simulink model "sampleModel1599_1"  (R2023a)
settings: Solver=VariableStepAuto  StartTime=0.0  StopTime=10.0  RelTol=1e-3
libraries: hdlsllib x2, simulink x2
settings Model: Creator=user1  LastModifiedBy=user1

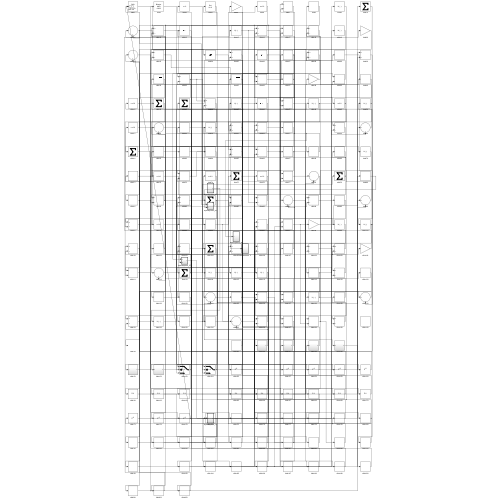
[thumbnail: Simulink's stored preview of the top-level diagram]
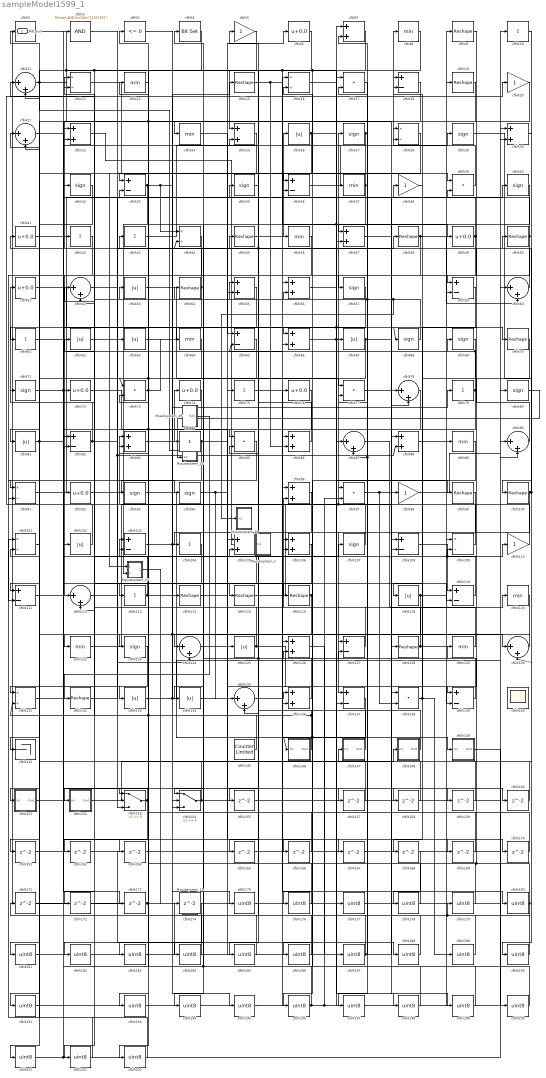
== system sampleModel1599_1 ==
  Mysubsystem_11 : Subsystem  TreatAsAtomicUnit=on  RTWFcnName=Mysubsystem_11
      settings: RTWFcnNameOpts=User specified  RTWFileNameOpts=Use function name
  Mysubsystem_2 : Subsystem  TreatAsAtomicUnit=on  RTWFcnName=Mysubsystem_2
      settings: RTWFcnNameOpts=User specified  RTWFileNameOpts=Use function name
  Mysubsystem_20 : Subsystem  TreatAsAtomicUnit=on  RTWFcnName=Mysubsystem_20
      settings: RTWFcnNameOpts=User specified  RTWFileNameOpts=Use function name
  Mysubsystem_27 : Subsystem  TreatAsAtomicUnit=on  RTWFcnName=Mysubsystem_27
      settings: RTWFcnNameOpts=User specified  RTWFileNameOpts=Use function name
  Mysubsystem_48 : Subsystem  TreatAsAtomicUnit=on  RTWFcnName=Mysubsystem_48
      settings: RTWFcnNameOpts=User specified  RTWFileNameOpts=Use function name
  Mysubsystem_49 : Subsystem  TreatAsAtomicUnit=on  RTWFcnName=Mysubsystem_49
      settings: RTWFcnNameOpts=User specified  RTWFileNameOpts=Use function name
  cfblk1 : ArithShift  BitShiftNumber=8
  cfblk{10,42..43,61,75,79,84,104,113} (9 alike) : Sum  Inputs=+  OutDataTypeStr=uint8
  cfblk{9,15,19,45,48,50,54,70,99..100,114..116,128,132} (15 alike) : Reshape
  cfblk{12,16,28,44,91,101,109,131} (8 alike) : Product  Inputs=*/  OutDataTypeStr=uint8  RndMeth=Zero  SaturateOnIntegerOverflow=on
  cfblk{26,53,62..63,67,81,102,118,125,133..134} (11 alike) : Abs  OutDataTypeStr=uint8  SaturateOnIntegerOverflow=off
  cfblk{18,33,36,59,65,82,103,108,111,119,127,137,139} (13 alike) : Sum  Inputs=+-  OutDataTypeStr=uint8
  cfblk{7,22,25,30,47,55..56,66,83,86,88,96,105..106,126,136} (16 alike) : Sum  OutDataTypeStr=uint8
  cfblk{27,29,32,35,40,57,68..69,71,80,93..94,107,123} (14 alike) : Signum
  cfblk{11,21,52,60,78,87,90,112,124,130,135} (11 alike) : Sum  Inputs=|++  OutDataTypeStr=uint8
  cfblk{5,20,38,98,110} (5 alike) : Gain  OutDataTypeStr=uint8
  cfblk{8,13,24,37,46,64,89,120,122,129} (10 alike) : MinMax  OutDataTypeStr=uint8
  cfblk{17,39,73,77,85,97,138} (7 alike) : DotProduct  OutDataTypeStr=uint8
  cfblk140 : Scope
      settings: Floating=on
  cfblk141 : Terminator
  cfblk145 : hdlsllib/Sources/Counter Limited  uplimit=7  tsamp=-1
  cfblk146 : Subsystem
      settings: LibrarySourceBlock=|
      | hdlsllib/Ports &
      | Subsystems/Subsystem
  cfblk147 : Subsystem
      settings: LibrarySourceBlock=|
      | hdlsllib/Ports &
      | Subsystems/Subsystem
  cfblk148 : Subsystem
      settings: LibrarySourceBlock=|
      | hdlsllib/Ports &
      | Subsystems/Subsystem
  cfblk149 : Subsystem
      settings: LibrarySourceBlock=|
      | hdlsllib/Ports &
      | Subsystems/Subsystem
  cfblk151 : Subsystem
      settings: LibrarySourceBlock=|
      | hdlsllib/Ports &
      | Subsystems/Subsystem
  cfblk152 : Subsystem
      settings: LibrarySourceBlock=|
      | hdlsllib/Ports &
      | Subsystems/Subsystem
  cfblk153 : Switch  OutDataTypeStr=uint8  SaturateOnIntegerOverflow=off  InputSameDT=off
  cfblk154 : Switch  OutDataTypeStr=uint8  SaturateOnIntegerOverflow=off  InputSameDT=off
  cfblk{155,157..163,165..174} (18 alike) : Delay  SampleTime=1
  cfblk{175..191,193..203} (28 alike) : DataTypeConversion  OutDataTypeStr=uint8  SaturateOnIntegerOverflow=off  RndMeth=Floor
  cfblk2 : simulink/Logic and Bit Operations/Bitwise Operator  logicop=AND  UseBitMask=on  BitMask=bin2dec('11011001')  BitMaskRealWorld=Stored Integer
      settings: LibrarySourceBlock=|
      | hdlsllib/Logic and Bit
      | Operations/Bitwise
      | Operator
  cfblk3 : hdlsllib/Logic and Bit Operations/Compare To Zero  relop=<=  OutDataTypeStr=uint8
  cfblk4 : simulink/Logic and Bit Operations/Bit Set  iBit=0
      settings: LibrarySourceBlock=|
      | hdlsllib/Logic and Bit
      | Operations/Bit Set
  cfblk{6,41,49,51,72,74,76,92} (8 alike) : Bias  Bias=0.0  SaturateOnIntegerOverflow=off
  Hdl_out : Outport  OutDataTypeStr=uint8
  wires:
  cfblk63/1 -> cfblk66/1
  cfblk68/1 -> Mysubsystem_48/1(In1), cfblk11/1, cfblk37/1
  cfblk59/1 -> cfblk118/1
  cfblk90/1 -> cfblk41/1
  cfblk87/1 -> cfblk120/1
  cfblk29/1 -> cfblk147/1(In1)
  cfblk102/1 -> cfblk20/1
  cfblk93/1 -> cfblk149/1(In1)
  cfblk97/1 -> cfblk98/1, cfblk138/2
  cfblk153/1 -> cfblk152/1(In1), cfblk162/1
  cfblk107/1 -> cfblk27/1, cfblk32/1
  cfblk91/1 -> cfblk38/1
  cfblk7/1 -> cfblk36/1, cfblk155/1
  cfblk40/1 -> cfblk47/2, cfblk183/1
  cfblk94/1 -> cfblk135/1, cfblk6/1
  cfblk122/1 -> cfblk97/1
  cfblk81/1 -> cfblk119/2, cfblk191/1
  cfblk89/1 -> cfblk196/1
  cfblk39/1 -> cfblk8/1
  cfblk136/1 -> cfblk103/1, cfblk85/2
  cfblk48/1 -> cfblk112/1, cfblk60/2
  cfblk10/1 -> cfblk100/1
  cfblk99/1 -> cfblk137/1
  cfblk41/1 -> cfblk24/1
  cfblk109/1 -> cfblk83/1
  cfblk154/1 -> cfblk90/2, cfblk21/2
  cfblk92/1 -> cfblk94/1
  cfblk130/1 -> cfblk124/1
  cfblk65/1 -> cfblk113/1
  cfblk36/1 -> cfblk28/1
  cfblk152/1(Out1) -> cfblk148/1(In1)
  cfblk103/1 -> cfblk127/1, cfblk195/1
  cfblk27/1 -> cfblk87/2, cfblk197/1, cfblk85/1
  cfblk54/1 -> cfblk42/1, cfblk153/2
  cfblk56/1 -> cfblk198/1
  cfblk138/1 -> cfblk18/1, cfblk189/1
  cfblk146/1(Out1) -> cfblk22/2, cfblk131/2
  cfblk11/1 -> Mysubsystem_20/1(In1), cfblk128/1
  cfblk84/1 -> cfblk111/2, cfblk158/1
  cfblk82/1 -> cfblk51/1, cfblk160/1
  cfblk1/1 -> cfblk63/1, cfblk87/1
  cfblk67/1 -> cfblk72/1, cfblk169/1
  cfblk45/1 -> cfblk26/1
  cfblk25/1 -> cfblk61/1
  cfblk37/1 -> cfblk33/1, cfblk134/1
  cfblk32/1 -> cfblk141/1
  cfblk57/1 -> cfblk92/1
  cfblk12/1 -> cfblk114/1
  cfblk76/1 -> cfblk133/1
  cfblk125/1 -> cfblk71/1, cfblk139/2
  cfblk33/1 -> Mysubsystem_27/2(In2), cfblk44/1, cfblk116/1
  cfblk110/1 -> cfblk21/1
  cfblk66/1 -> cfblk29/1, cfblk68/1, cfblk130/1
  cfblk116/1 -> cfblk176/1, cfblk194/1
  cfblk132/1 -> cfblk88/2, cfblk48/1
  cfblk88/1 -> cfblk40/1
  cfblk151/1(Out1) -> cfblk107/1
  cfblk74/1 -> cfblk123/1, cfblk202/1
  cfblk43/1 -> cfblk7/1
  cfblk98/1 -> cfblk60/1
  cfblk148/1(Out1) -> cfblk55/1
  cfblk50/1 -> cfblk12/1, cfblk153/3
  cfblk38/1 -> cfblk18/2
  cfblk79/1 -> cfblk154/1, cfblk69/1
  cfblk75/1 -> cfblk180/1
  cfblk55/1 -> cfblk91/1
  cfblk112/1 -> cfblk35/1
  cfblk2/1 -> cfblk39/1
  cfblk100/1 -> cfblk146/1(In1), cfblk186/1, cfblk130/2, cfblk50/1
  cfblk104/1 -> cfblk112/2
  cfblk123/1 -> cfblk151/1(In1)
  cfblk83/1 -> cfblk74/1
  cfblk62/1 -> cfblk154/2
  cfblk134/1 -> cfblk137/2
  cfblk72/1 -> cfblk125/1
  cfblk17/1 -> cfblk57/1
  cfblk35/1 -> cfblk115/1
  cfblk49/1 -> cfblk28/2, cfblk55/2
  cfblk139/1 -> cfblk93/1
  cfblk6/1 -> cfblk122/1, cfblk36/2
  cfblk5/1 -> cfblk25/1
  cfblk135/1 -> cfblk136/1
  cfblk69/1 -> cfblk65/2, cfblk168/1
  cfblk115/1 -> cfblk78/2
  cfblk30/1 -> cfblk190/1
  cfblk101/1 -> cfblk201/1
  cfblk86/1 -> cfblk45/1
  cfblk108/1 -> cfblk119/1
  cfblk133/1 -> cfblk80/1, cfblk79/1
  cfblk145/1 -> cfblk62/1, cfblk73/2
  cfblk96/1 -> cfblk104/1
  cfblk61/1 -> cfblk102/1
  cfblk147/1(Out1) -> cfblk5/1, cfblk44/2
  cfblk78/1 -> cfblk108/2
  cfblk70/1 -> cfblk139/1
  cfblk120/1 -> cfblk131/1
  cfblk127/1 -> cfblk96/2
  cfblk9/1 -> cfblk59/1
  cfblk20/1 -> cfblk81/1, cfblk203/1
  cfblk21/1 -> cfblk70/1
  cfblk8/1 -> cfblk82/1, cfblk11/2
  cfblk44/1 -> cfblk91/2
  cfblk71/1 -> cfblk46/1, cfblk170/1
  cfblk129/1 -> cfblk7/2
  cfblk51/1 -> cfblk84/1
  cfblk52/1 -> cfblk124/2
  cfblk18/1 -> cfblk82/2
  cfblk128/1 -> cfblk19/1, cfblk13/1
  cfblk15/1 -> cfblk49/1, cfblk86/2
  cfblk118/1 -> cfblk154/3, cfblk181/1, cfblk110/1
  cfblk53/1 -> cfblk77/1
  cfblk73/1 -> cfblk33/2, cfblk64/1
  cfblk64/1 -> cfblk111/1
  cfblk4/1 -> cfblk153/1, cfblk73/1
  cfblk19/1 -> cfblk47/1
  cfblk77/1 -> cfblk39/2
  cfblk113/1 -> cfblk15/1, cfblk52/1
  cfblk60/1 -> cfblk12/2
  cfblk126/1 -> cfblk187/1
  cfblk119/1 -> cfblk109/2, cfblk52/2
  cfblk24/1 -> cfblk65/1
  cfblk26/1 -> cfblk99/1, cfblk165/1
  cfblk155/1 -> cfblk66/2
  cfblk114/1 -> cfblk157/1
  cfblk157/1 -> cfblk1/1
  cfblk158/1 -> cfblk127/2
  cfblk111/1 -> cfblk159/1
  cfblk159/1 -> cfblk103/2
  cfblk160/1 -> cfblk25/2
  cfblk42/1 -> cfblk161/1
  cfblk161/1 -> cfblk108/1
  cfblk13/1 -> cfblk163/1
  cfblk163/1 -> cfblk78/1
  cfblk165/1 -> cfblk136/2
  cfblk137/1 -> cfblk166/1
  cfblk166/1 -> cfblk135/2
  cfblk124/1 -> cfblk167/1
  cfblk167/1 -> cfblk90/1
  cfblk169/1 -> cfblk17/1
  cfblk170/1 -> cfblk83/2
  cfblk171/1 -> cfblk59/2
  cfblk85/1 -> cfblk172/1
  cfblk172/1 -> cfblk96/1
  cfblk131/1 -> cfblk173/1
  cfblk173/1 -> cfblk109/1, Hdl_out/1
  cfblk3/1 -> cfblk175/1
  cfblk175/1 -> cfblk76/1
  cfblk176/1 -> cfblk3/1
  cfblk16/1 -> cfblk177/1
  cfblk177/1 -> cfblk17/2
  cfblk168/1 -> cfblk178/1
  cfblk178/1 -> cfblk16/1
  cfblk179/1 -> cfblk16/2
  cfblk180/1 -> cfblk129/1, cfblk4/1, cfblk171/1
  cfblk181/1 -> cfblk75/1
  cfblk174/1 -> cfblk182/1
  cfblk182/1 -> cfblk88/1
  cfblk183/1 -> cfblk174/1
  cfblk105/1 -> cfblk184/1
  cfblk184/1 -> cfblk53/1
  cfblk46/1 -> cfblk185/1
  cfblk185/1 -> cfblk105/1
  cfblk186/1 -> cfblk105/2
  cfblk187/1 -> cfblk86/1, cfblk77/2
  cfblk162/1 -> cfblk188/1
  cfblk188/1 -> cfblk126/1
  cfblk189/1 -> cfblk126/2
  cfblk190/1 -> cfblk179/1, cfblk138/1
  cfblk191/1 -> cfblk30/1
  cfblk106/1 -> cfblk193/1
  cfblk193/1 -> cfblk67/1
  cfblk194/1 -> cfblk106/1
  cfblk195/1 -> cfblk106/2
  cfblk196/1 -> cfblk9/1, cfblk97/2, cfblk43/1
  cfblk197/1 -> cfblk89/1
  cfblk198/1 -> cfblk54/1, cfblk22/1
  cfblk47/1 -> cfblk199/1
  cfblk199/1 -> cfblk56/1
  cfblk149/1(Out1) -> cfblk200/1
  cfblk200/1 -> cfblk56/2
  cfblk201/1 -> cfblk2/1, cfblk10/1
  cfblk202/1 -> cfblk101/1
  cfblk203/1 -> cfblk101/2
  cfblk22/1 -> Mysubsystem_2/1(In1)
  Mysubsystem_11/1(Out1) -> cfblk30/2
  cfblk80/1 -> Mysubsystem_20/2(In2)
  cfblk28/1 -> Mysubsystem_27/1(In1)
  Mysubsystem_27/1(Out1) -> Mysubsystem_11/1(In1)
  Mysubsystem_49/1(Out1) -> cfblk132/1

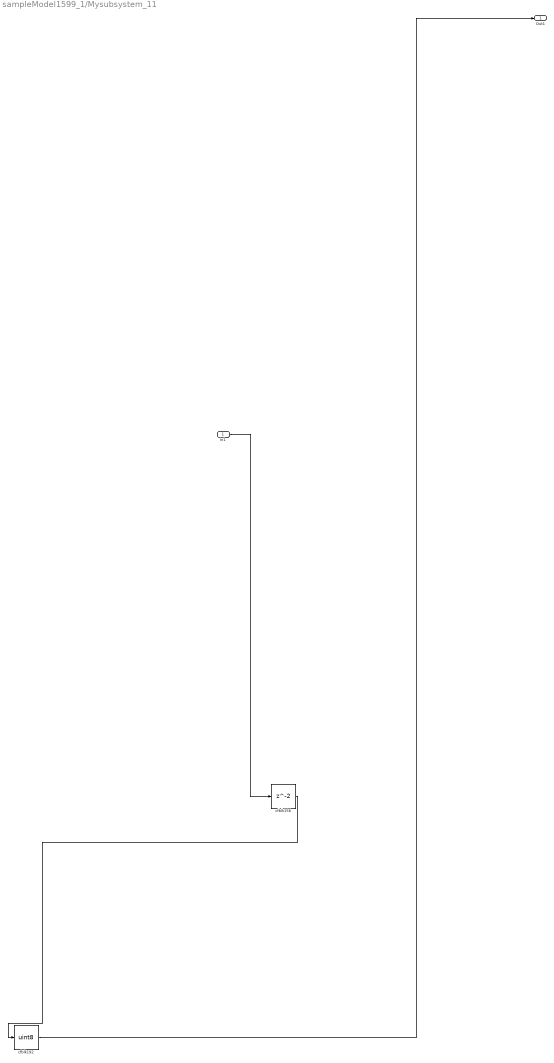
== system sampleModel1599_1/Mysubsystem_11 ==
  In1 : Inport
  cfblk156 : Delay  SampleTime=1
  cfblk192 : DataTypeConversion  OutDataTypeStr=uint8  SaturateOnIntegerOverflow=off  RndMeth=Floor
  Out1 : Outport
  wires:
  cfblk192/1 -> Out1/1
  cfblk156/1 -> cfblk192/1
  In1/1 -> cfblk156/1

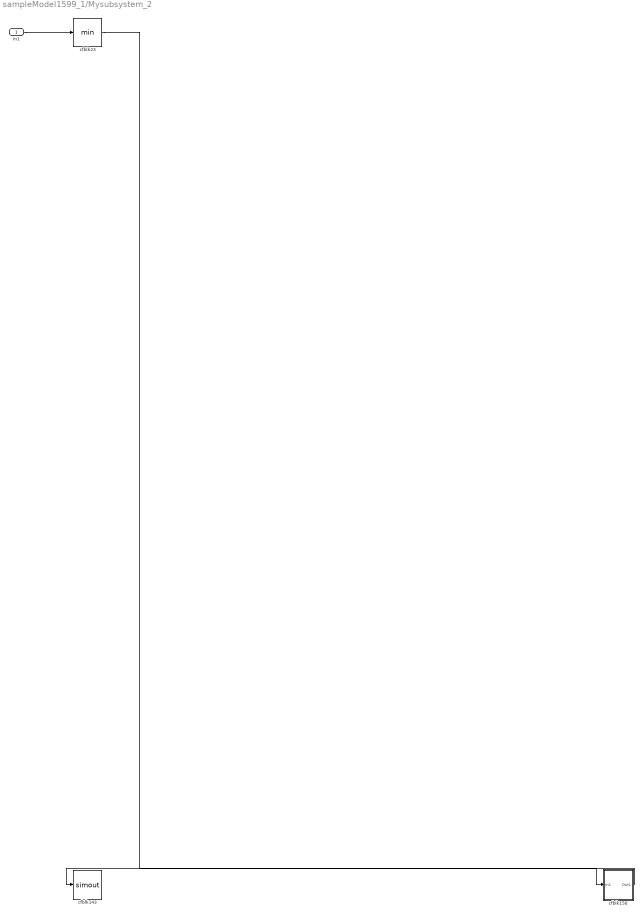
== system sampleModel1599_1/Mysubsystem_2 ==
  In1 : Inport
  cfblk143 : ToWorkspace  VariableName=simout  SaveFormat=Timeseries  SampleTime=-1
  cfblk150 : Subsystem
      settings: LibrarySourceBlock=|
      | hdlsllib/Ports &
      | Subsystems/Subsystem
  cfblk23 : MinMax
  wires:
  cfblk150/1(Out1) -> cfblk143/1
  In1/1 -> cfblk23/1
  cfblk23/1 -> cfblk150/1(In1)

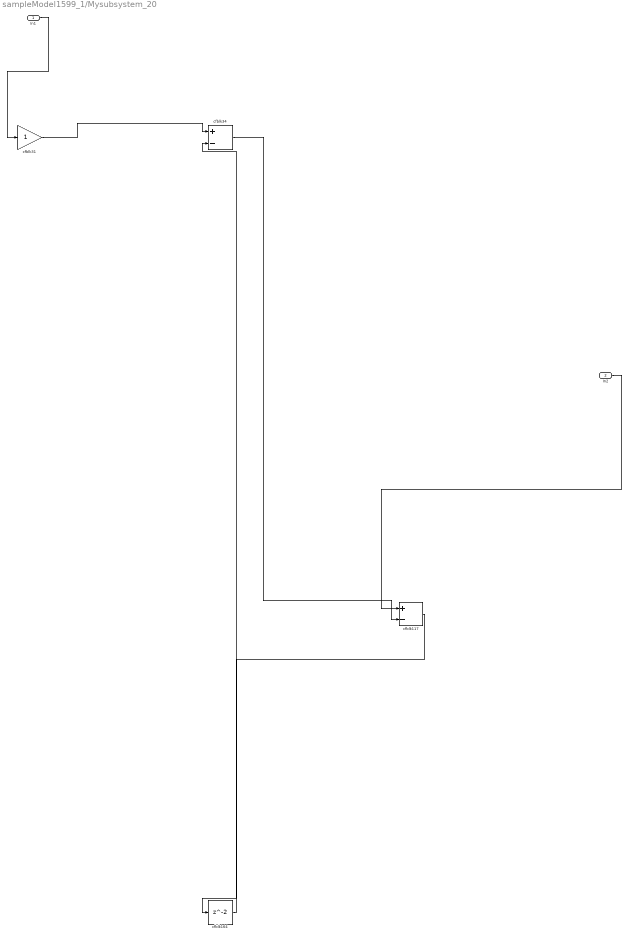
== system sampleModel1599_1/Mysubsystem_20 ==
  In1 : Inport
  In2 : Inport  Port=2
  cfblk117 : Sum  Inputs=+-
  cfblk164 : Delay  SampleTime=1
  cfblk31 : Gain
  cfblk34 : Sum  Inputs=+-
  wires:
  cfblk164/1 -> cfblk34/2
  In1/1 -> cfblk31/1
  cfblk31/1 -> cfblk34/1
  cfblk117/1 -> cfblk164/1
  cfblk34/1 -> cfblk117/2
  In2/1 -> cfblk117/1

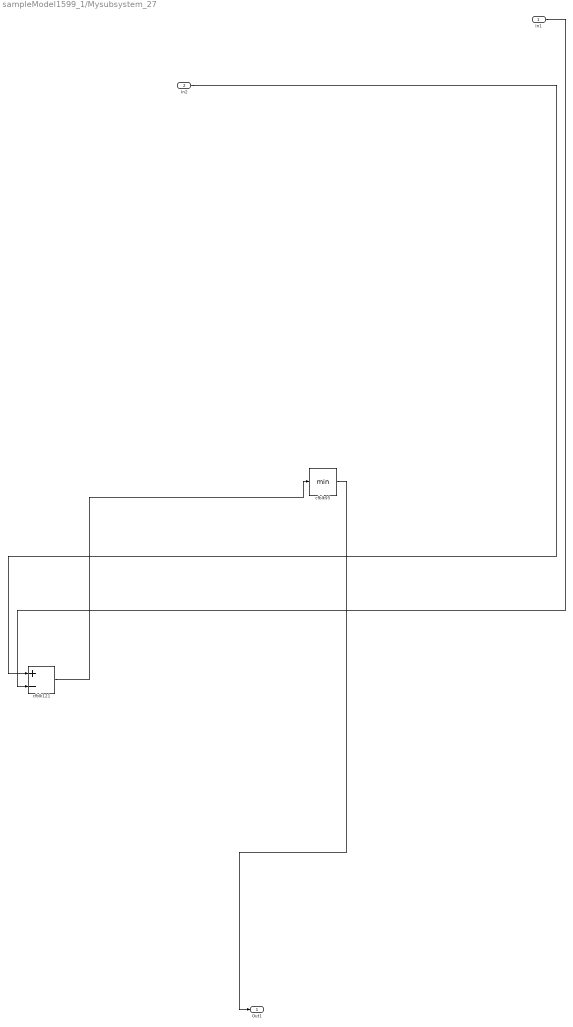
== system sampleModel1599_1/Mysubsystem_27 ==
  In1 : Inport
  In2 : Inport  Port=2
  cfblk121 : Sum  Inputs=+-
  cfblk95 : MinMax
  Out1 : Outport
  wires:
  cfblk95/1 -> Out1/1
  cfblk121/1 -> cfblk95/1
  In1/1 -> cfblk121/2
  In2/1 -> cfblk121/1

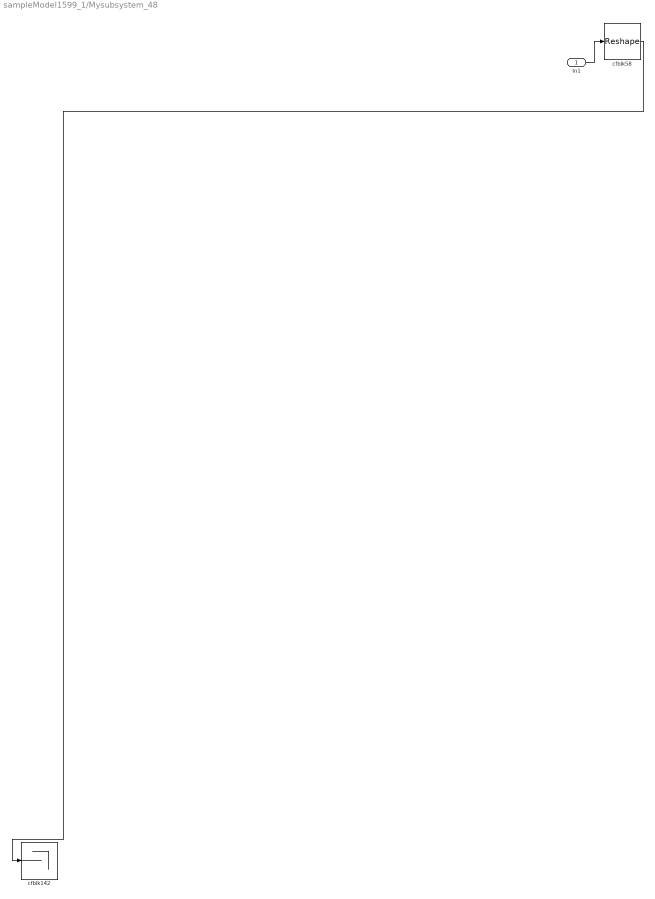
== system sampleModel1599_1/Mysubsystem_48 ==
  In1 : Inport
  cfblk142 : Terminator
  cfblk58 : Reshape
  wires:
  cfblk58/1 -> cfblk142/1
  In1/1 -> cfblk58/1

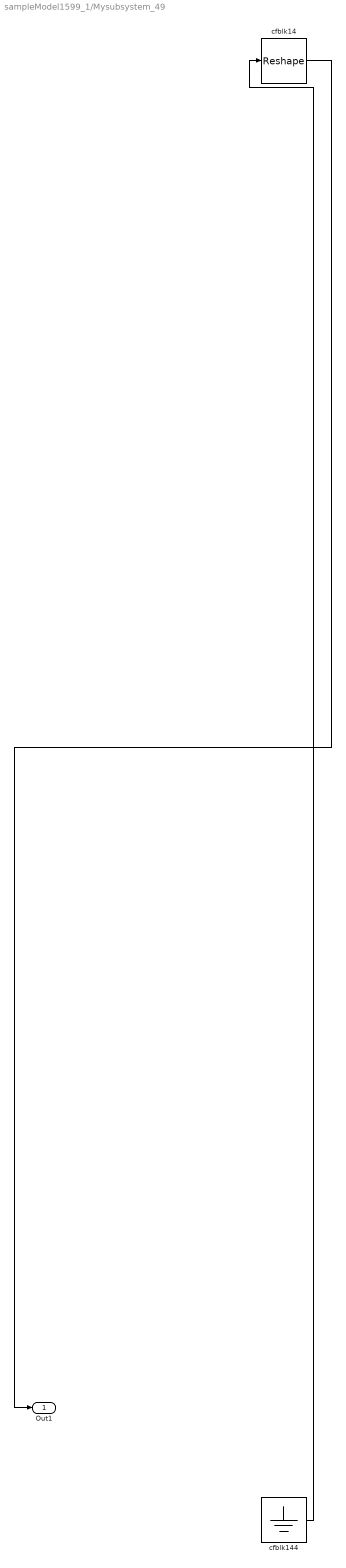
== system sampleModel1599_1/Mysubsystem_49 ==
  cfblk14 : Reshape
  cfblk144 : Ground
  Out1 : Outport
  wires:
  cfblk144/1 -> cfblk14/1
  cfblk14/1 -> Out1/1

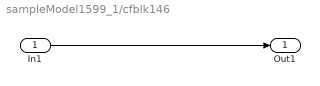
== system sampleModel1599_1/cfblk146 ==
  In1 : Inport
  Out1 : Outport
  wires:
  In1/1 -> Out1/1

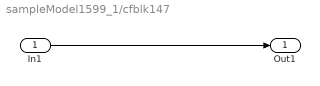
== system sampleModel1599_1/cfblk147 ==
  In1 : Inport
  Out1 : Outport
  wires:
  In1/1 -> Out1/1

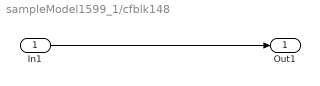
== system sampleModel1599_1/cfblk148 ==
  In1 : Inport
  Out1 : Outport
  wires:
  In1/1 -> Out1/1

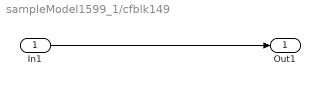
== system sampleModel1599_1/cfblk149 ==
  In1 : Inport
  Out1 : Outport
  wires:
  In1/1 -> Out1/1

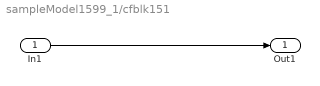
== system sampleModel1599_1/cfblk151 ==
  In1 : Inport
  Out1 : Outport
  wires:
  In1/1 -> Out1/1

== system sampleModel1599_1/cfblk152 ==
  In1 : Inport
  Out1 : Outport
  wires:
  In1/1 -> Out1/1

== system sampleModel1599_1/Mysubsystem_2/cfblk150 ==
  In1 : Inport
  Out1 : Outport
  wires:
  In1/1 -> Out1/1
